simulink model "sistema_fisico_completo"  (R2023b)
settings: Solver=VariableStepAuto  StartTime=0.0  StopTime=10.0  RelTol=1e-3
undefined symbols (not defined in the file): b_cx, b_cy, b_hb, b_hEb, b_hwu, b_t, b_tb, b_tw, bh_eq, bt_eq, CI, g, H_c, i_h, i_t, Jh_eq, Jt_eq, K_cy, K_hwu, K_tw, L_h0, M_s, m_t, r_hd, r_td, T_hb_max, T_hEb_max, T_tb_max, Y_t0
settings Model: Creator=Ferran  LastModifiedBy=Ferran

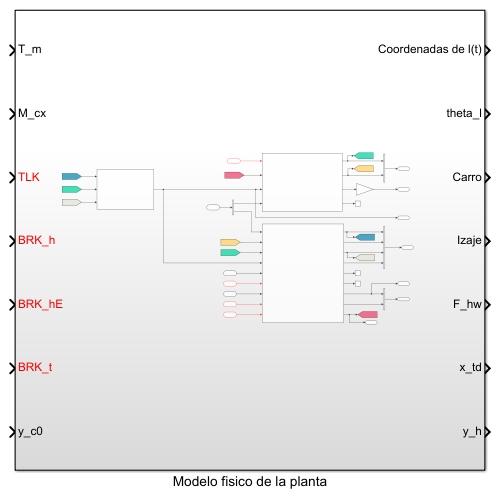
[thumbnail: Simulink's stored preview of the top-level diagram]
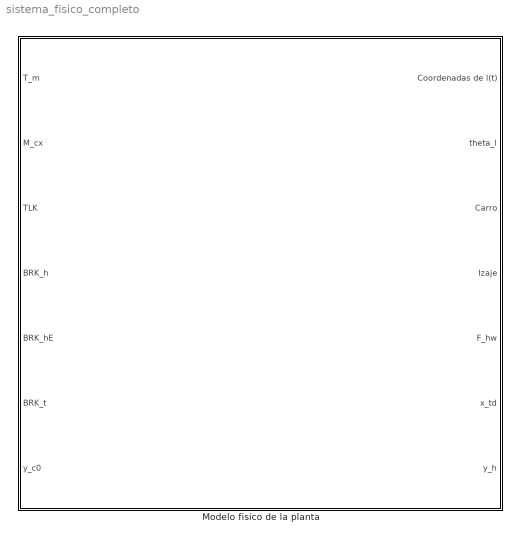
== system sistema_fisico_completo ==
  Modelo fisico de la planta : Subsystem

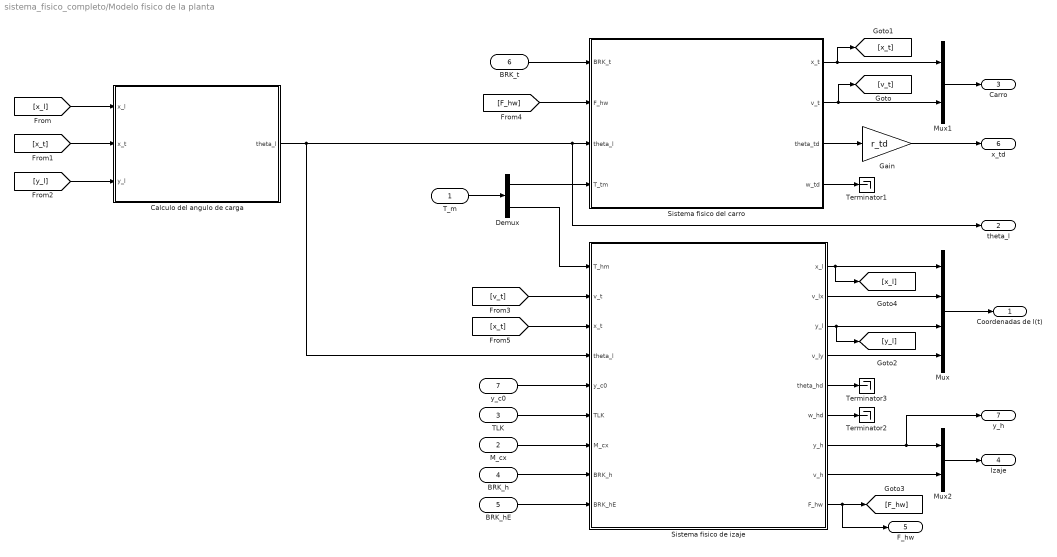
== system sistema_fisico_completo/Modelo fisico de la planta ==
  T_m : Inport
  M_cx : Inport  Port=2
  TLK : Inport  Port=3
  BRK_h : Inport  Port=4
  BRK_hE : Inport  Port=5
  BRK_t : Inport  Port=6
  y_c0 : Inport  Port=7
  Calculo del angulo de carga : Subsystem
  Demux : Demux  Outputs=2
  Gain : Gain  Gain=r_td
  Mux : Mux
  Mux1 : Mux  Inputs=2
  Mux2 : Mux  Inputs=2
  Sistema fisico de izaje : Subsystem
  Sistema fisico del carro : Subsystem
  Terminator1 : Terminator
  Terminator2 : Terminator
  Terminator3 : Terminator
  Coordenadas de l(t) : Outport
  theta_l : Outport  Port=2
  Carro : Outport  Port=3
  Izaje : Outport  Port=4
  F_hw : Outport  Port=5
  x_td : Outport  Port=6
  y_h : Outport  Port=7
  wires:
  [x_l] -> Calculo del angulo de carga/1(x_l)
  Sistema fisico del carro/3(theta_td) -> Gain/1
  Calculo del angulo de carga/1(theta_l) -> Sistema fisico del carro/3(theta_l), theta_l/1, Sistema fisico de izaje/4(theta_l)
  Sistema fisico de izaje/2(v_lx) -> Mux/2
  [x_t] -> Calculo del angulo de carga/2(x_t)
  y_c0/1 -> Sistema fisico de izaje/5(y_c0)
  Sistema fisico del carro/1(x_t) -> Mux1/1, [x_t]
  Sistema fisico de izaje/1(x_l) -> Mux/1, [x_l]
  Sistema fisico del carro/4(w_td) -> Terminator1/1
  [y_l] -> Calculo del angulo de carga/3(y_l)
  Sistema fisico de izaje/3(y_l) -> Mux/3, [y_l]
  [v_t] -> Sistema fisico de izaje/2(v_t)
  [x_t] -> Sistema fisico de izaje/3(x_t)
  Sistema fisico del carro/2(v_t) -> Mux1/2, [v_t]
  BRK_hE/1 -> Sistema fisico de izaje/9(BRK_hE)
  M_cx/1 -> Sistema fisico de izaje/7(M_cx)
  BRK_h/1 -> Sistema fisico de izaje/8(BRK_h)
  TLK/1 -> Sistema fisico de izaje/6(TLK)
  Demux/2 -> Sistema fisico de izaje/1(T_hm)
  [F_hw] -> Sistema fisico del carro/2(F_hw)
  Sistema fisico de izaje/9(F_hw) -> F_hw/1, [F_hw]
  Sistema fisico de izaje/4(v_ly) -> Mux/4
  Mux/1 -> Coordenadas de l(t)/1
  Mux1/1 -> Carro/1
  Sistema fisico de izaje/8(v_h) -> Mux2/2
  Mux2/1 -> Izaje/1
  Sistema fisico de izaje/5(theta_hd) -> Terminator3/1
  Sistema fisico de izaje/6(w_hd) -> Terminator2/1
  BRK_t/1 -> Sistema fisico del carro/1(BRK_t)
  Demux/1 -> Sistema fisico del carro/4(T_tm)
  T_m/1 -> Demux/1
  Sistema fisico de izaje/7(y_h) -> y_h/1, Mux2/1
  Gain/1 -> x_td/1

== system sistema_fisico_completo/Modelo fisico de la planta/Calculo del angulo de carga ==
  x_l : Inport
  x_t : Inport  Port=2
  y_l : Inport  Port=3
  Atan2 : Trigonometry  Operator=atan2
  Constant : Constant  Value=Y_t0
  Sum : Sum  Inputs=+-
  Sum1 : Sum  Inputs=+-
  theta_l : Outport
  wires:
  x_t/1 -> Sum/2
  Sum1/1 -> Atan2/2
  x_l/1 -> Sum/1
  Sum/1 -> Atan2/1
  Atan2/1 -> theta_l/1
  y_l/1 -> Sum1/2
  Constant/1 -> Sum1/1

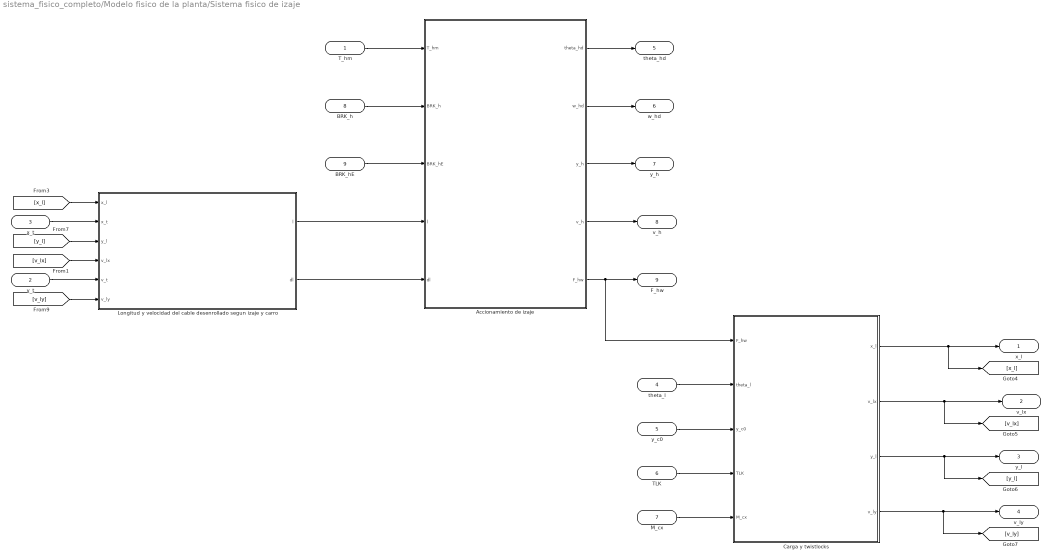
== system sistema_fisico_completo/Modelo fisico de la planta/Sistema fisico de izaje ==
  T_hm : Inport
  v_t : Inport  Port=2
  x_t : Inport  Port=3
  theta_l : Inport  Port=4
  y_c0 : Inport  Port=5
  TLK : Inport  Port=6
  M_cx : Inport  Port=7
  BRK_h : Inport  Port=8
  BRK_hE : Inport  Port=9
  Accionamiento de izaje : Subsystem
  Carga y twistlocks : Subsystem
  Longitud y velocidad del cable desenrollado segun izaje y carro : Subsystem
  x_l : Outport
  v_lx : Outport  Port=2
  y_l : Outport  Port=3
  v_ly : Outport  Port=4
  theta_hd : Outport  Port=5
  w_hd : Outport  Port=6
  y_h : Outport  Port=7
  v_h : Outport  Port=8
  F_hw : Outport  Port=9
  wires:
  [y_l] -> Longitud y velocidad del cable desenrollado segun izaje y carro/3(y_l)
  Accionamiento de izaje/5(F_hw) -> F_hw/1, Carga y twistlocks/1(F_hw)
  BRK_hE/1 -> Accionamiento de izaje/3(BRK_hE)
  Carga y twistlocks/1(x_l) -> x_l/1, [x_l]
  Carga y twistlocks/4(v_ly) -> v_ly/1, [v_ly]
  Accionamiento de izaje/3(y_h) -> y_h/1
  Carga y twistlocks/2(v_lx) -> v_lx/1, [v_lx]
  Longitud y velocidad del cable desenrollado segun izaje y carro/1(l) -> Accionamiento de izaje/4(l)
  Carga y twistlocks/3(y_l) -> y_l/1, [y_l]
  [v_lx] -> Longitud y velocidad del cable desenrollado segun izaje y carro/4(v_lx)
  [v_ly] -> Longitud y velocidad del cable desenrollado segun izaje y carro/6(v_ly)
  TLK/1 -> Carga y twistlocks/4(TLK)
  [x_l] -> Longitud y velocidad del cable desenrollado segun izaje y carro/1(x_l)
  T_hm/1 -> Accionamiento de izaje/1(T_hm)
  Accionamiento de izaje/1(theta_hd) -> theta_hd/1
  y_c0/1 -> Carga y twistlocks/3(y_c0)
  BRK_h/1 -> Accionamiento de izaje/2(BRK_h)
  Longitud y velocidad del cable desenrollado segun izaje y carro/2(dl) -> Accionamiento de izaje/5(dl)
  v_t/1 -> Longitud y velocidad del cable desenrollado segun izaje y carro/5(v_t)
  Accionamiento de izaje/4(v_h) -> v_h/1
  theta_l/1 -> Carga y twistlocks/2(theta_l)
  Accionamiento de izaje/2(w_hd) -> w_hd/1
  M_cx/1 -> Carga y twistlocks/5(M_cx)
  x_t/1 -> Longitud y velocidad del cable desenrollado segun izaje y carro/2(x_t)

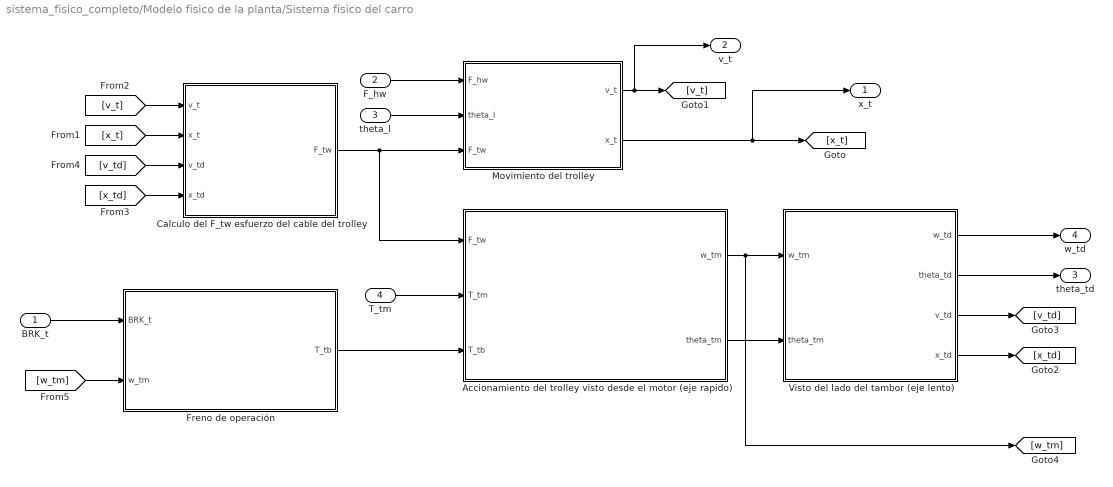
== system sistema_fisico_completo/Modelo fisico de la planta/Sistema fisico del carro ==
  BRK_t : Inport
  F_hw : Inport  Port=2
  theta_l : Inport  Port=3
  T_tm : Inport  Port=4
  Accionamiento del trolley visto desde el motor (eje rapido) : Subsystem
  Calculo del F_tw esfuerzo del cable del trolley : Subsystem
  Freno de operación : Subsystem
  Movimiento del trolley : Subsystem
  Visto del lado del tambor (eje lento) : Subsystem
  x_t : Outport
  v_t : Outport  Port=2
  theta_td : Outport  Port=3
  w_td : Outport  Port=4
  wires:
  [v_t] -> Calculo del F_tw esfuerzo del cable del trolley/1(v_t)
  Visto del lado del tambor (eje lento)/3(v_td) -> [v_td]
  Freno de operación/1(T_tb) -> Accionamiento del trolley visto desde el motor (eje rapido)/3(T_tb)
  Movimiento del trolley/1(v_t) -> v_t/1, [v_t]
  Movimiento del trolley/2(x_t) -> x_t/1, [x_t]
  Visto del lado del tambor (eje lento)/2(theta_td) -> theta_td/1
  BRK_t/1 -> Freno de operación/1(BRK_t)
  [w_tm] -> Freno de operación/2(w_tm)
  Accionamiento del trolley visto desde el motor (eje rapido)/1(w_tm) -> [w_tm], Visto del lado del tambor (eje lento)/1(w_tm)
  [x_td] -> Calculo del F_tw esfuerzo del cable del trolley/4(x_td)
  Accionamiento del trolley visto desde el motor (eje rapido)/2(theta_tm) -> Visto del lado del tambor (eje lento)/2(theta_tm)
  [x_t] -> Calculo del F_tw esfuerzo del cable del trolley/2(x_t)
  [v_td] -> Calculo del F_tw esfuerzo del cable del trolley/3(v_td)
  theta_l/1 -> Movimiento del trolley/2(theta_l)
  Visto del lado del tambor (eje lento)/4(x_td) -> [x_td]
  T_tm/1 -> Accionamiento del trolley visto desde el motor (eje rapido)/2(T_tm)
  Calculo del F_tw esfuerzo del cable del trolley/1(F_tw) -> Accionamiento del trolley visto desde el motor (eje rapido)/1(F_tw), Movimiento del trolley/3(F_tw)
  F_hw/1 -> Movimiento del trolley/1(F_hw)
  Visto del lado del tambor (eje lento)/1(w_td) -> w_td/1

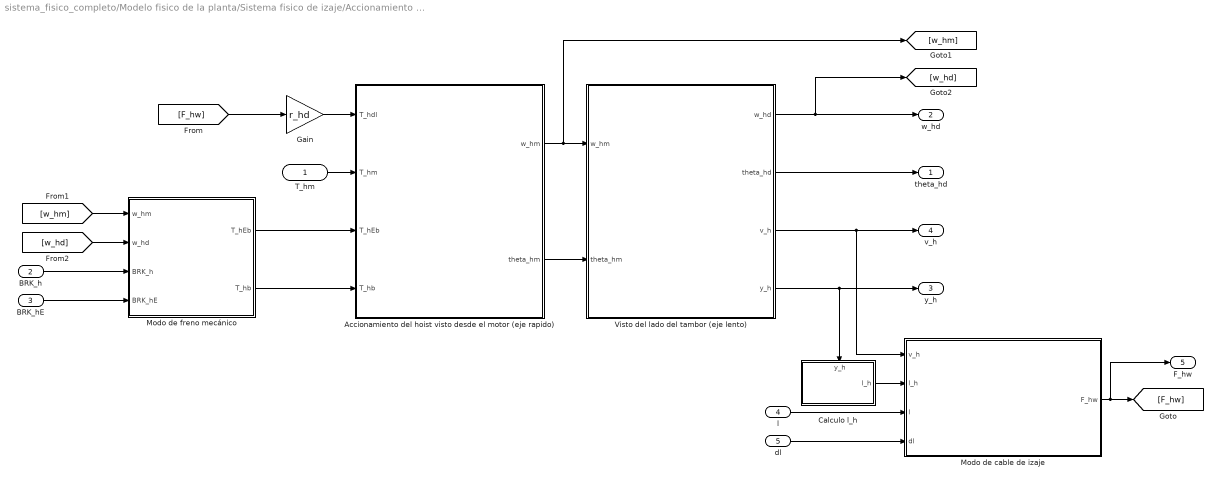
== system sistema_fisico_completo/Modelo fisico de la planta/Sistema fisico de izaje/Accionamiento de izaje ==
  T_hm : Inport
  BRK_h : Inport  Port=2
  BRK_hE : Inport  Port=3
  l : Inport  Port=4
  dl : Inport  Port=5
  Accionamiento del hoist visto desde el motor (eje rapido) : Subsystem
  Calculo l_h : Subsystem
      settings: PortSchema="{\"entries\":[{\"content\":{\"sides\":[{\"content\":{\"connectorIds\":[\"Out1\"]},\"type\":\"ConnectorPlacement.EquallySpacedRectSide\",\"uuid\":\"07ea2d8b-a4bd-4a00-9f3e-d3723522cead\"},{\"content\":{\"side\":\"RIGHT\"},\"type\":\"ConnectorPlacement.EquallySpacedRectSide\",\"uuid\":\"e7371649-c13b-4c3e-a52c-6db8f2f471a9\"},{\"content\":{\"side\":\"TOP\"},\"type\":\"ConnectorPlacement.EquallySpacedRectSide\",\"uuid\":\"bf44ddc9-8ab8-43a2-b974-62ce3b2d20dc\"},{\"content\":{\"connectorIds\":[\"In1\"],\"side\":\"BOTTOM\"},\"type\":\"ConnectorPlacement.EquallySpacedRectSide\",\"uuid\":\"68df679a-1ec0-4ce0-a9ee-39677e661654\"}]},\"type\":\"ConnectorPlacement.EquallySpacedConnector\",\"uuid\":\"345e5710-5df9-4bf4-96c9-62f27951d1e0\"}],\"packageUris\":[\"http://schema.mathworks.com/mf0/Connector/R2020b\"],\"version\":\"1.0\"}"
  Gain : Gain  Gain=r_hd
  Modo de cable de izaje : Subsystem
  Modo de freno mecánico : Subsystem
  Visto del lado del tambor (eje lento) : Subsystem
  theta_hd : Outport
  w_hd : Outport  Port=2
  y_h : Outport  Port=3
  v_h : Outport  Port=4
  F_hw : Outport  Port=5
  wires:
  Gain/1 -> Accionamiento del hoist visto desde el motor (eje rapido)/1(T_hdl)
  Accionamiento del hoist visto desde el motor (eje rapido)/1(w_hm) -> Visto del lado del tambor (eje lento)/1(w_hm), [w_hm]
  Visto del lado del tambor (eje lento)/1(w_hd) -> w_hd/1, [w_hd]
  Accionamiento del hoist visto desde el motor (eje rapido)/2(theta_hm) -> Visto del lado del tambor (eje lento)/2(theta_hm)
  dl/1 -> Modo de cable de izaje/4(dl)
  l/1 -> Modo de cable de izaje/3(l)
  [F_hw] -> Gain/1
  BRK_hE/1 -> Modo de freno mecánico/4(BRK_hE)
  Visto del lado del tambor (eje lento)/4(y_h) -> y_h/1, Calculo l_h/1(y_h)
  BRK_h/1 -> Modo de freno mecánico/3(BRK_h)
  Visto del lado del tambor (eje lento)/3(v_h) -> v_h/1, Modo de cable de izaje/1(v_h)
  Visto del lado del tambor (eje lento)/2(theta_hd) -> theta_hd/1
  T_hm/1 -> Accionamiento del hoist visto desde el motor (eje rapido)/2(T_hm)
  [w_hd] -> Modo de freno mecánico/2(w_hd)
  [w_hm] -> Modo de freno mecánico/1(w_hm)
  Calculo l_h/1(l_h) -> Modo de cable de izaje/2(l_h)
  Modo de freno mecánico/2(T_hb) -> Accionamiento del hoist visto desde el motor (eje rapido)/4(T_hb)
  Modo de cable de izaje/1(F_hw) -> F_hw/1, [F_hw]
  Modo de freno mecánico/1(T_hEb) -> Accionamiento del hoist visto desde el motor (eje rapido)/3(T_hEb)

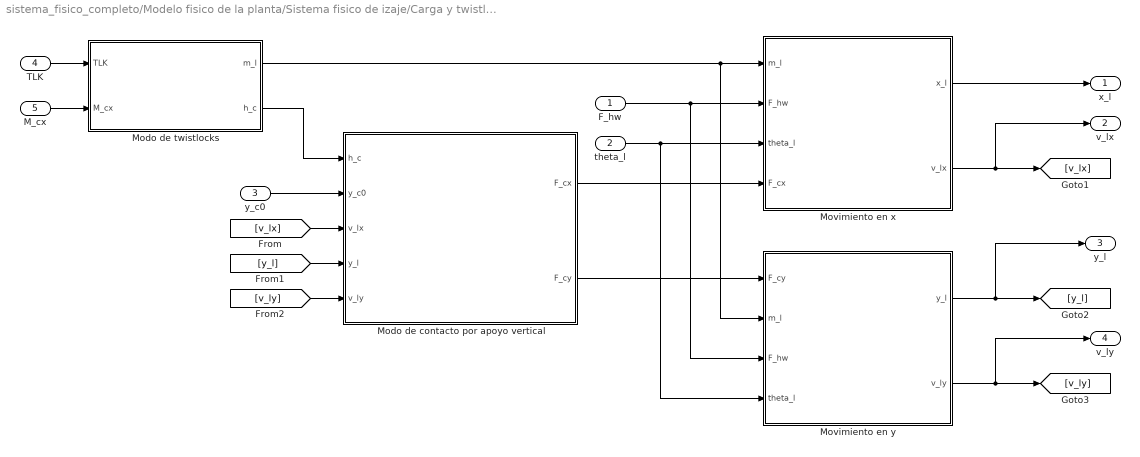
== system sistema_fisico_completo/Modelo fisico de la planta/Sistema fisico de izaje/Carga y twistlocks ==
  F_hw : Inport
  theta_l : Inport  Port=2
  y_c0 : Inport  Port=3
  TLK : Inport  Port=4
  M_cx : Inport  Port=5
  Modo de contacto por apoyo vertical : Subsystem
  Modo de twistlocks : Subsystem
  Movimiento en x : Subsystem
  Movimiento en y : Subsystem
  x_l : Outport
  v_lx : Outport  Port=2
  y_l : Outport  Port=3
  v_ly : Outport  Port=4
  wires:
  theta_l/1 -> Movimiento en y/4(theta_l), Movimiento en x/3(theta_l)
  Movimiento en y/2(v_ly) -> v_ly/1, [v_ly]
  y_c0/1 -> Modo de contacto por apoyo vertical/2(y_c0)
  Modo de contacto por apoyo vertical/2(F_cy) -> Movimiento en y/1(F_cy)
  [y_l] -> Modo de contacto por apoyo vertical/4(y_l)
  [v_lx] -> Modo de contacto por apoyo vertical/3(v_lx)
  Movimiento en x/2(v_lx) -> v_lx/1, [v_lx]
  TLK/1 -> Modo de twistlocks/1(TLK)
  Movimiento en x/1(x_l) -> x_l/1
  Modo de twistlocks/1(m_l) -> Movimiento en x/1(m_l), Movimiento en y/2(m_l)
  [v_ly] -> Modo de contacto por apoyo vertical/5(v_ly)
  Movimiento en y/1(y_l) -> y_l/1, [y_l]
  Modo de contacto por apoyo vertical/1(F_cx) -> Movimiento en x/4(F_cx)
  F_hw/1 -> Movimiento en y/3(F_hw), Movimiento en x/2(F_hw)
  M_cx/1 -> Modo de twistlocks/2(M_cx)
  Modo de twistlocks/2(h_c) -> Modo de contacto por apoyo vertical/1(h_c)

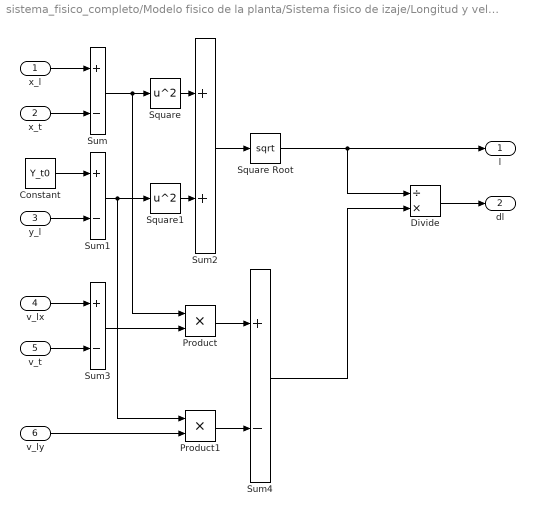
== system sistema_fisico_completo/Modelo fisico de la planta/Sistema fisico de izaje/Longitud y velocidad del cable desenrollado segun izaje y carro ==
  x_l : Inport
  x_t : Inport  Port=2
  y_l : Inport  Port=3
  v_lx : Inport  Port=4
  v_t : Inport  Port=5
  v_ly : Inport  Port=6
  Constant : Constant  Value=Y_t0
  Divide : Product  Inputs=/*
  Product : Product
  Product1 : Product
  Square : Math  Operator=square
  Square Root : Sqrt
  Square1 : Math  Operator=square
  Sum{,1,3..4} (4 alike) : Sum  Inputs=+-
  Sum2 : Sum
  l : Outport
  dl : Outport  Port=2
  wires:
  Sum/1 -> Product/1, Square/1
  Divide/1 -> dl/1
  Product1/1 -> Sum4/2
  Sum3/1 -> Product/2
  Product/1 -> Sum4/1
  Square Root/1 -> l/1, Divide/1
  Constant/1 -> Sum1/1
  Sum4/1 -> Divide/2
  y_l/1 -> Sum1/2
  x_l/1 -> Sum/1
  Square1/1 -> Sum2/2
  v_t/1 -> Sum3/2
  Sum1/1 -> Square1/1, Product1/1
  v_ly/1 -> Product1/2
  Square/1 -> Sum2/1
  v_lx/1 -> Sum3/1
  x_t/1 -> Sum/2
  Sum2/1 -> Square Root/1

== system sistema_fisico_completo/Modelo fisico de la planta/Sistema fisico del carro/Accionamiento del trolley visto desde el motor (eje rapido) ==
  F_tw : Inport
  T_tm : Inport  Port=2
  T_tb : Inport  Port=3
  Gain : Gain  Gain=r_td / i_t
  Integrator : Integrator  InitialCondition=CI(1) * (i_t / r_td)
  Integrator1 : Integrator
  Momento de inercia del trolley equivalente : Gain  Gain=1 / Jt_eq
  Sum : Sum  Inputs=--++
  Viscosidad del trolley equivalente : Gain  Gain=bt_eq
  w_tm : Outport
  theta_tm : Outport  Port=2
  wires:
  Gain/1 -> Sum/2
  Integrator/1 -> theta_tm/1
  Sum/1 -> Momento de inercia del trolley equivalente/1
  Integrator1/1 -> Viscosidad del trolley equivalente/1, w_tm/1, Integrator/1  "w_tm"
  Viscosidad del trolley equivalente/1 -> Sum/1
  Momento de inercia del trolley equivalente/1 -> Integrator1/1  "dw_tm"
  F_tw/1 -> Gain/1
  T_tb/1 -> Sum/4
  T_tm/1 -> Sum/3

== system sistema_fisico_completo/Modelo fisico de la planta/Sistema fisico del carro/Calculo del F_tw esfuerzo del cable del trolley ==
  v_t : Inport
  x_t : Inport  Port=2
  v_td : Inport  Port=3
  x_td : Inport  Port=4
  Gain : Gain  Gain=K_tw
  Gain1 : Gain  Gain=b_tw
  Sum : Sum  Inputs=+-
  Sum2 : Sum  Inputs=+-
  Sum3 : Sum
  F_tw : Outport
  wires:
  x_td/1 -> Sum/1
  Sum/1 -> Gain/1
  v_td/1 -> Sum2/1
  Sum2/1 -> Gain1/1
  v_t/1 -> Sum2/2
  x_t/1 -> Sum/2
  Sum3/1 -> F_tw/1
  Gain/1 -> Sum3/1
  Gain1/1 -> Sum3/2

== system sistema_fisico_completo/Modelo fisico de la planta/Sistema fisico del carro/Freno de operación ==
  note: Si BRK_t = 0 (Off - desenergizado) ... entonces ... T_tb != 0
      | Si BRK_t = 1 (On - energizado) ... entonces ... T_tb == 0
  BRK_t : Inport
  w_tm : Inport  Port=2
  Constant1 : Constant  Value=-T_tb_max
  Constant2 : Constant  Value=T_tb_max
  Flip : Subsystem
  Gain : Gain  Gain=- b_tb
  Max : MinMax  Function=max  Inputs=2
  Min : MinMax  Inputs=2
  Product : Product
  T_tb : Outport
  wires:
  Constant1/1 -> Max/1
  w_tm/1 -> Gain/1
  Max/1 -> Min/2
  BRK_t/1 -> Flip/1(BRK_t)
  Min/1 -> Product/2
  Product/1 -> T_tb/1
  Constant2/1 -> Min/1
  Gain/1 -> Max/2
  Flip/1(Out1) -> Product/1

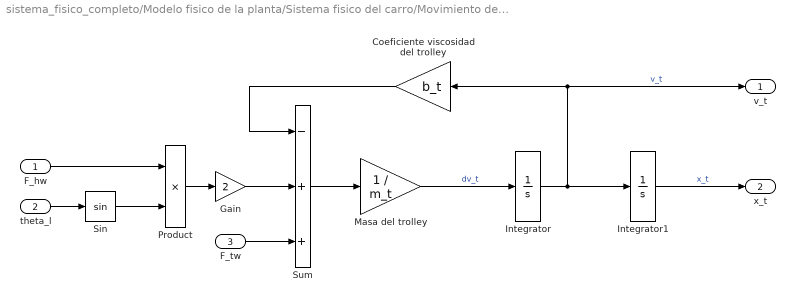
== system sistema_fisico_completo/Modelo fisico de la planta/Sistema fisico del carro/Movimiento del trolley ==
  F_hw : Inport
  theta_l : Inport  Port=2
  F_tw : Inport  Port=3
  Coeficiente viscosidad del trolley : Gain  Gain=b_t
  Gain : Gain  Gain=2
  Integrator : Integrator
  Integrator1 : Integrator  InitialCondition=CI(1)
  Masa del trolley : Gain  Gain=1 / m_t
  Product : Product
  Sin : Trigonometry
  Sum : Sum  Inputs=-++
  v_t : Outport
  x_t : Outport  Port=2
  wires:
  Sin/1 -> Product/2
  F_tw/1 -> Sum/3
  Integrator/1 -> v_t/1, Coeficiente viscosidad del trolley/1, Integrator1/1  "v_t"
  F_hw/1 -> Product/1
  Integrator1/1 -> x_t/1  "x_t"
  Product/1 -> Gain/1
  Sum/1 -> Masa del trolley/1
  theta_l/1 -> Sin/1
  Masa del trolley/1 -> Integrator/1  "dv_t"
  Gain/1 -> Sum/2
  Coeficiente viscosidad del trolley/1 -> Sum/1

== system sistema_fisico_completo/Modelo fisico de la planta/Sistema fisico del carro/Visto del lado del tambor (eje lento) ==
  w_tm : Inport
  theta_tm : Inport  Port=2
  Gain : Gain  Gain=1 / i_t
  Gain1 : Gain  Gain=1 / i_t
  r_td : Gain  Gain=r_td
  r_td1 : Gain  Gain=r_td
  w_td : Outport
  theta_td : Outport  Port=2
  v_td : Outport  Port=3
  x_td : Outport  Port=4
  wires:
  Gain1/1 -> r_td1/1, theta_td/1
  Gain/1 -> w_td/1, r_td/1
  w_tm/1 -> Gain/1
  theta_tm/1 -> Gain1/1
  r_td/1 -> v_td/1
  r_td1/1 -> x_td/1

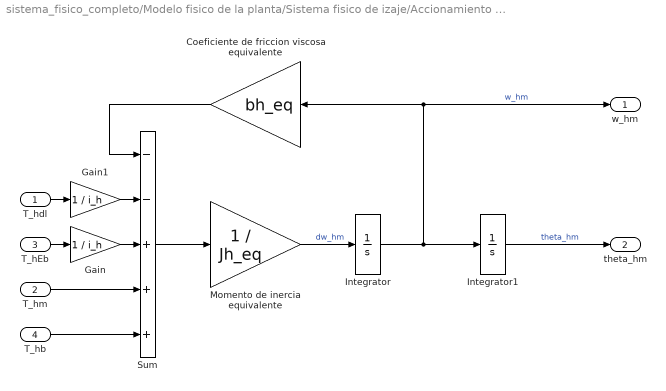
== system sistema_fisico_completo/Modelo fisico de la planta/Sistema fisico de izaje/Accionamiento de izaje/Accionamiento del hoist visto desde el motor (eje rapido) ==
  T_hdl : Inport
  T_hm : Inport  Port=2
  T_hEb : Inport  Port=3
  T_hb : Inport  Port=4
  Coeficiente de friccion viscosa equivalente : Gain  Gain=bh_eq
  Gain : Gain  Gain=1 / i_h
  Gain1 : Gain  Gain=1 / i_h
  Integrator : Integrator
  Integrator1 : Integrator  InitialCondition=CI(3) * ((2 * i_h)/ r_hd)
  Momento de inercia equivalente : Gain  Gain=1 / Jh_eq
  Sum : Sum  Inputs=--+++
  w_hm : Outport
  theta_hm : Outport  Port=2
  wires:
  Integrator1/1 -> theta_hm/1  "theta_hm"
  Coeficiente de friccion viscosa equivalente/1 -> Sum/1
  T_hm/1 -> Sum/4
  Momento de inercia equivalente/1 -> Integrator/1  "dw_hm"
  T_hEb/1 -> Gain/1
  Integrator/1 -> Coeficiente de friccion viscosa equivalente/1, w_hm/1, Integrator1/1  "w_hm"
  T_hb/1 -> Sum/5
  Sum/1 -> Momento de inercia equivalente/1
  T_hdl/1 -> Gain1/1
  Gain/1 -> Sum/3
  Gain1/1 -> Sum/2

== system sistema_fisico_completo/Modelo fisico de la planta/Sistema fisico de izaje/Accionamiento de izaje/Calculo l_h ==
  y_h : Inport
  Constant : Constant  Value=Y_t0
  Sum : Sum  Inputs=+-
  l_h : Outport
  wires:
  Constant/1 -> Sum/1
  Sum/1 -> l_h/1
  y_h/1 -> Sum/2

== system sistema_fisico_completo/Modelo fisico de la planta/Sistema fisico de izaje/Accionamiento de izaje/Modo de cable de izaje ==
  note: El bloque if analiza cual bloque de accion se habilita (action subsystem), luego se usa el bloque merge para unir las salidas y determinar la salida final segun se haya decidido desde el bloque if
      |
      | En este caso el modo de cable:
      | cuando l(t) >= l_h(t) entonces esta tensado
      | cuando l(t) < l_h(t) entonces esta flojo
  v_h : Inport
  l_h : Inport  Port=2
  l : Inport  Port=3
  dl : Inport  Port=4
  Cable flojo : Subsystem  TreatAsAtomicUnit=on
  Cable tensado : Subsystem  TreatAsAtomicUnit=on
  Decision del modo de cable de izaje : If  NumInputs=2  IfExpression=u2 >= u1
  Merge : Merge
  F_hw : Outport
  wires:
  Decision del modo de cable de izaje/1 -> Cable tensado/Action
  Decision del modo de cable de izaje/2 -> Cable flojo/Action
  l/1 -> Decision del modo de cable de izaje/2, Cable tensado/2(l)
  Cable flojo/1(Out1) -> Merge/2
  dl/1 -> Cable tensado/4(dl)
  l_h/1 -> Decision del modo de cable de izaje/1, Cable tensado/1(l_h)
  Cable tensado/1(F_hw) -> Merge/1
  v_h/1 -> Cable tensado/3(v_h)
  Merge/1 -> F_hw/1

== system sistema_fisico_completo/Modelo fisico de la planta/Sistema fisico de izaje/Accionamiento de izaje/Modo de freno mecánico ==
  w_hm : Inport
  w_hd : Inport  Port=2
  BRK_h : Inport  Port=3
  BRK_hE : Inport  Port=4
  Freno de emergencia : Subsystem
  Freno de operación : Subsystem
  T_hEb : Outport
  T_hb : Outport  Port=2
  wires:
  w_hm/1 -> Freno de operación/2(w_hm)
  BRK_hE/1 -> Freno de emergencia/1(BRK_hE)
  Freno de operación/1(T_hb) -> T_hb/1
  Freno de emergencia/1(T_hEb) -> T_hEb/1
  w_hd/1 -> Freno de emergencia/2(w_hd)
  BRK_h/1 -> Freno de operación/1(BRK_h)

== system sistema_fisico_completo/Modelo fisico de la planta/Sistema fisico de izaje/Accionamiento de izaje/Visto del lado del tambor (eje lento) ==
  w_hm : Inport
  theta_hm : Inport  Port=2
  Gain : Gain  Gain=1 / i_h
  Gain1 : Gain  Gain=1 / i_h
  r_td : Gain  Gain=r_hd / 2
  r_td1 : Gain  Gain=r_hd / 2
  w_hd : Outport
  theta_hd : Outport  Port=2
  v_h : Outport  Port=3
  y_h : Outport  Port=4
  wires:
  Gain1/1 -> r_td1/1, theta_hd/1
  Gain/1 -> w_hd/1, r_td/1
  w_hm/1 -> Gain/1
  theta_hm/1 -> Gain1/1
  r_td/1 -> v_h/1
  r_td1/1 -> y_h/1

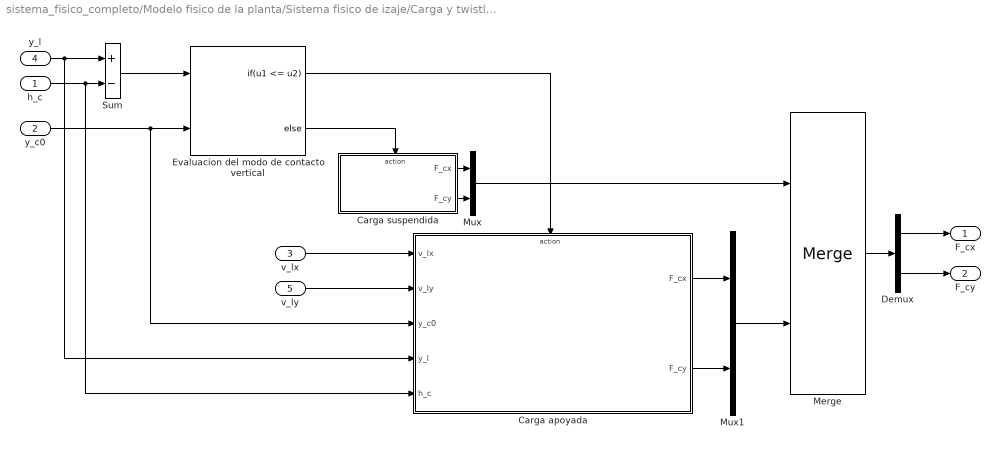
== system sistema_fisico_completo/Modelo fisico de la planta/Sistema fisico de izaje/Carga y twistlocks/Modo de contacto por apoyo vertical ==
  h_c : Inport
  y_c0 : Inport  Port=2
  v_lx : Inport  Port=3
  y_l : Inport  Port=4
  v_ly : Inport  Port=5
  Carga apoyada : Subsystem  TreatAsAtomicUnit=on
  Carga suspendida : Subsystem  TreatAsAtomicUnit=on
  Demux : Demux  Outputs=2
  Evaluacion del modo de contacto vertical : If  NumInputs=2  IfExpression=u1 <= u2
  Merge : Merge
  Mux : Mux  Inputs=2
  Mux1 : Mux  Inputs=2
  Sum : Sum  Inputs=+-
  F_cx : Outport
  F_cy : Outport  Port=2
  wires:
  Carga apoyada/2(F_cy) -> Mux1/2
  Evaluacion del modo de contacto vertical/1 -> Carga apoyada/Action
  Evaluacion del modo de contacto vertical/2 -> Carga suspendida/Action
  y_c0/1 -> Carga apoyada/3(y_c0), Evaluacion del modo de contacto vertical/2
  v_lx/1 -> Carga apoyada/1(v_lx)
  Sum/1 -> Evaluacion del modo de contacto vertical/1
  y_l/1 -> Carga apoyada/4(y_l), Sum/1
  h_c/1 -> Sum/2, Carga apoyada/5(h_c)
  Carga suspendida/1(F_cx) -> Mux/1
  Carga suspendida/2(F_cy) -> Mux/2
  Mux/1 -> Merge/1
  Carga apoyada/1(F_cx) -> Mux1/1
  Mux1/1 -> Merge/2
  Merge/1 -> Demux/1
  Demux/1 -> F_cx/1
  Demux/2 -> F_cy/1
  v_ly/1 -> Carga apoyada/2(v_ly)

== system sistema_fisico_completo/Modelo fisico de la planta/Sistema fisico de izaje/Carga y twistlocks/Modo de twistlocks ==
  note: Si TLK = 0 (Off) ... entonces ... h_c = 0
      | Si TLK = 1 (On) ... entonces ... h_c = H_c
  note: Si TLK = 0 (Off) ... entonces ... m_l = M_s
      | Si TLK = 1 (On) ... entonces ... m_l = M_s + M_cx
  TLK : Inport
  M_cx : Inport  Port=2
  Altura del container : Constant  Value=H_c
  Masa del spreader : Constant  Value=M_s
  Product : Product
  Product1 : Product
  Sum : Sum
  m_l : Outport
  h_c : Outport  Port=2
  wires:
  M_cx/1 -> Product/2
  Sum/1 -> m_l/1
  TLK/1 -> Product/1, Product1/1
  Masa del spreader/1 -> Sum/1
  Product/1 -> Sum/2
  Altura del container/1 -> Product1/2
  Product1/1 -> h_c/1

== system sistema_fisico_completo/Modelo fisico de la planta/Sistema fisico de izaje/Carga y twistlocks/Movimiento en x ==
  m_l : Inport
  F_hw : Inport  Port=2
  theta_l : Inport  Port=3
  F_cx : Inport  Port=4
  Divide : Product  Inputs=*/
  Gain : Gain  Gain=2
  Integrator : Integrator
  Integrator1 : Integrator
  Product : Product
  Sin : Trigonometry
  Sum : Sum  Inputs=-+
  x_l : Outport
  v_lx : Outport  Port=2
  wires:
  Integrator1/1 -> x_l/1
  Product/1 -> Sum/1
  Sum/1 -> Divide/1
  m_l/1 -> Divide/2
  Integrator/1 -> v_lx/1, Integrator1/1  "dx_l"
  Sin/1 -> Product/1
  theta_l/1 -> Sin/1
  F_cx/1 -> Sum/2
  Divide/1 -> Integrator/1  "ddx_l"
  F_hw/1 -> Gain/1
  Gain/1 -> Product/2

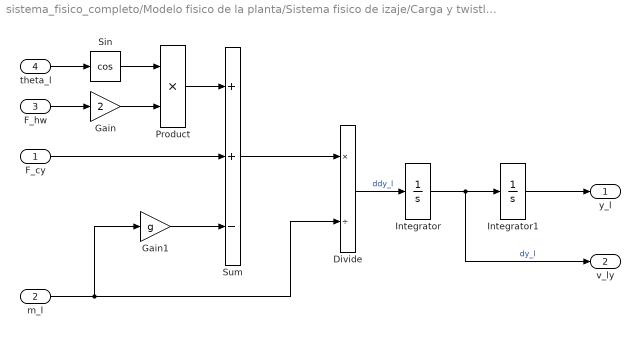
== system sistema_fisico_completo/Modelo fisico de la planta/Sistema fisico de izaje/Carga y twistlocks/Movimiento en y ==
  F_cy : Inport
  m_l : Inport  Port=2
  F_hw : Inport  Port=3
  theta_l : Inport  Port=4
  Divide : Product  Inputs=*/
  Gain : Gain  Gain=2
  Gain1 : Gain  Gain=g
  Integrator : Integrator
  Integrator1 : Integrator  InitialCondition=CI(3)
  Product : Product
  Sin : Trigonometry  Operator=cos
  Sum : Sum  Inputs=++-
  y_l : Outport
  v_ly : Outport  Port=2
  wires:
  Integrator1/1 -> y_l/1
  Product/1 -> Sum/1
  Sum/1 -> Divide/1
  m_l/1 -> Divide/2, Gain1/1
  Integrator/1 -> v_ly/1, Integrator1/1  "dy_l"
  Sin/1 -> Product/1
  theta_l/1 -> Sin/1
  F_cy/1 -> Sum/2
  Divide/1 -> Integrator/1  "ddy_l"
  F_hw/1 -> Gain/1
  Gain/1 -> Product/2
  Gain1/1 -> Sum/3

== system sistema_fisico_completo/Modelo fisico de la planta/Sistema fisico del carro/Freno de operación/Flip ==
  note: Como la decision de desenergizar (Off) representa un 0 pero a la salida existe un valor diferente de cero, se utiliza este sistema para cambiar el cero (0) por un uno (1).
      |
      | Esto es debido a que se usa el bloque de producto que multiplica la señal de BRK_t por el calculo pertinente a T_tb.
  BRK_t : Inport
  Constant : Constant  Value=[1 0]
  Selector : Selector  IndexMode=Zero-based  InputPortWidth=2  IndexOptions=Starting index (port)  Indices=[1 3]  OutputSizes=1
  Out1 : Outport
  wires:
  BRK_t/1 -> Selector/2
  Constant/1 -> Selector/1
  Selector/1 -> Out1/1

== system sistema_fisico_completo/Modelo fisico de la planta/Sistema fisico de izaje/Accionamiento de izaje/Modo de cable de izaje/Cable flojo ==
  Action Port : ActionPort
  Zero : Constant  Value=0  OutDataTypeStr=Inherit: Inherit via back propagation
  Out1 : Outport
  wires:
  Zero/1 -> Out1/1

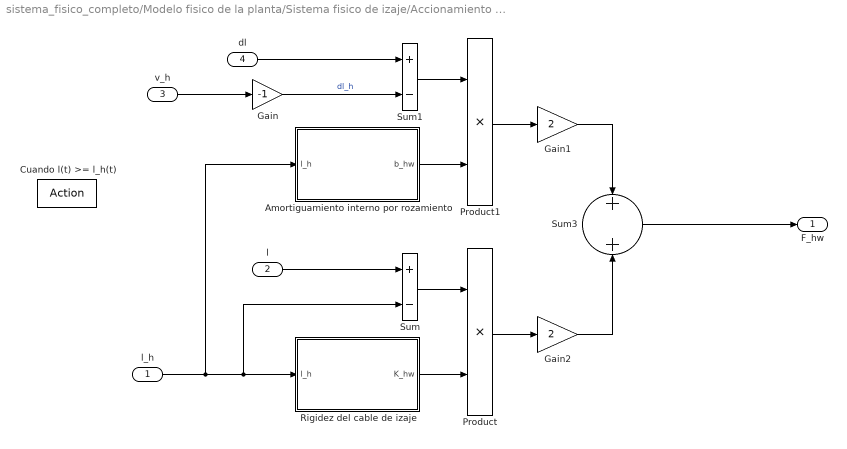
== system sistema_fisico_completo/Modelo fisico de la planta/Sistema fisico de izaje/Accionamiento de izaje/Modo de cable de izaje/Cable tensado ==
  l_h : Inport
  l : Inport  Port=2
  v_h : Inport  Port=3
  dl : Inport  Port=4
  Cuando l(t) >= l_h(t) : ActionPort
  Amortiguamiento interno por rozamiento : Subsystem
  Gain : Gain  Gain=-1
  Gain1 : Gain  Gain=2
  Gain2 : Gain  Gain=2
  Product : Product
  Product1 : Product
  Rigidez del cable de izaje : Subsystem
  Sum : Sum  Inputs=+-
  Sum1 : Sum  Inputs=+-
  Sum3 : Sum
  F_hw : Outport
  wires:
  l/1 -> Sum/1
  l_h/1 -> Amortiguamiento interno por rozamiento/1(l_h), Rigidez del cable de izaje/1(l_h), Sum/2
  Sum3/1 -> F_hw/1
  Gain1/1 -> Sum3/1
  Gain2/1 -> Sum3/2
  Rigidez del cable de izaje/1(K_hw) -> Product/2
  Amortiguamiento interno por rozamiento/1(b_hw) -> Product1/2
  Sum1/1 -> Product1/1
  Sum/1 -> Product/1
  v_h/1 -> Gain/1
  Product1/1 -> Gain1/1
  Product/1 -> Gain2/1
  dl/1 -> Sum1/1
  Gain/1 -> Sum1/2  "dl_h"

== system sistema_fisico_completo/Modelo fisico de la planta/Sistema fisico de izaje/Accionamiento de izaje/Modo de freno mecánico/Freno de emergencia ==
  note: Si BRK_h = 0 (Off - desenergizado) ... entonces ... T_hb != 0
      | Si BRK_h = 1 (On - energizado) ... entonces ... T_hb == 0
  BRK_hE : Inport
  w_hd : Inport  Port=2
  Flip : Subsystem
  Gain : Gain  Gain=- b_hEb
  Product : Product
  Saturation : Saturate  UpperLimit=T_hEb_max  LowerLimit=-T_hEb_max
  T_hEb : Outport
  wires:
  w_hd/1 -> Gain/1
  BRK_hE/1 -> Flip/1(BRK_hE)
  Product/1 -> T_hEb/1
  Gain/1 -> Saturation/1
  Flip/1(Out1) -> Product/1
  Saturation/1 -> Product/2

== system sistema_fisico_completo/Modelo fisico de la planta/Sistema fisico de izaje/Accionamiento de izaje/Modo de freno mecánico/Freno de operación ==
  note: Si BRK_h = 0 (Off - desenergizado) ... entonces ... T_hb != 0
      | Si BRK_h = 1 (On - energizado) ... entonces ... T_hb == 0
  BRK_h : Inport
  w_hm : Inport  Port=2
  Flip : Subsystem
  Gain : Gain  Gain=- b_hb
  Product : Product
  Saturation : Saturate  UpperLimit=T_hb_max  LowerLimit=-T_hb_max
  T_hb : Outport
  wires:
  w_hm/1 -> Gain/1
  BRK_h/1 -> Flip/1(BRK_h)
  Product/1 -> T_hb/1
  Flip/1(Out1) -> Product/1
  Saturation/1 -> Product/2
  Gain/1 -> Saturation/1

== system sistema_fisico_completo/Modelo fisico de la planta/Sistema fisico de izaje/Carga y twistlocks/Modo de contacto por apoyo vertical/Carga apoyada ==
  v_lx : Inport
  v_ly : Inport  Port=2
  y_c0 : Inport  Port=3
  y_l : Inport  Port=4
  h_c : Inport  Port=5
  Action Port : ActionPort
  Gain : Gain  Gain=- b_cx
  Gain1 : Gain  Gain=K_cy
  Gain2 : Gain  Gain=b_cy
  Sum : Sum  Inputs=+-
  Sum1 : Sum  Inputs=-++
  F_cx : Outport
  F_cy : Outport  Port=2
  wires:
  v_lx/1 -> Gain/1
  Gain/1 -> F_cx/1
  Gain1/1 -> Sum/1
  Sum/1 -> F_cy/1
  Gain2/1 -> Sum/2
  v_ly/1 -> Gain2/1
  Sum1/1 -> Gain1/1
  y_l/1 -> Sum1/1
  h_c/1 -> Sum1/2
  y_c0/1 -> Sum1/3

== system sistema_fisico_completo/Modelo fisico de la planta/Sistema fisico de izaje/Carga y twistlocks/Modo de contacto por apoyo vertical/Carga suspendida ==
  Action Port : ActionPort
  Zero : Constant  Value=0  OutDataTypeStr=Inherit: Inherit via back propagation
  F_cx : Outport
  F_cy : Outport  Port=2
  wires:
  Zero/1 -> F_cx/1, F_cy/1

== system sistema_fisico_completo/Modelo fisico de la planta/Sistema fisico de izaje/Accionamiento de izaje/Modo de cable de izaje/Cable tensado/Amortiguamiento interno por rozamiento ==
  l_h : Inport
  Constant : Constant  Value=L_h0
  Gain : Gain  Gain=2
  Gain1 : Gain  Gain=b_hwu
  Sum : Sum
  b_hw : Outport
  wires:
  Sum/1 -> Gain1/1
  Gain/1 -> Sum/1
  Gain1/1 -> b_hw/1
  Constant/1 -> Sum/2
  l_h/1 -> Gain/1

== system sistema_fisico_completo/Modelo fisico de la planta/Sistema fisico de izaje/Accionamiento de izaje/Modo de cable de izaje/Cable tensado/Rigidez del cable de izaje ==
  l_h : Inport
  Constant : Constant  Value=K_hwu
  Constant1 : Constant  Value=L_h0
  Divide : Product  Inputs=*/
  Gain : Gain  Gain=2
  Sum : Sum
  K_hw : Outport
  wires:
  Constant1/1 -> Sum/2
  Sum/1 -> Divide/2
  Gain/1 -> Sum/1
  Constant/1 -> Divide/1
  Divide/1 -> K_hw/1
  l_h/1 -> Gain/1

== system sistema_fisico_completo/Modelo fisico de la planta/Sistema fisico de izaje/Accionamiento de izaje/Modo de freno mecánico/Freno de emergencia/Flip ==
  note: Como la decision de desenergizar (Off) representa un 0 pero a la salida existe un valor diferente de cero, se utiliza este sistema para cambiar el cero (0) por un uno (1).
      |
      | Esto es debido a que se usa el bloque de producto que multiplica la señal de BRK_hE por el calculo pertinente a T_hEb.
  BRK_hE : Inport
  Constant : Constant  Value=[1 0]
  Selector : Selector  IndexMode=Zero-based  InputPortWidth=2  IndexOptions=Starting index (port)  Indices=[1 3]  OutputSizes=1
  Out1 : Outport
  wires:
  BRK_hE/1 -> Selector/2
  Constant/1 -> Selector/1
  Selector/1 -> Out1/1

== system sistema_fisico_completo/Modelo fisico de la planta/Sistema fisico de izaje/Accionamiento de izaje/Modo de freno mecánico/Freno de operación/Flip ==
  note: Como la decision de desenergizar (Off) representa un 0 pero a la salida existe un valor diferente de cero, se utiliza este sistema para cambiar el cero (0) por un uno (1).
      |
      | Esto es debido a que se usa el bloque de producto que multiplica la señal de BRK_h por el calculo pertinente a T_hb.
  BRK_h : Inport
  Constant : Constant  Value=[1 0]
  Selector : Selector  IndexMode=Zero-based  InputPortWidth=2  IndexOptions=Starting index (port)  Indices=[1 3]  OutputSizes=1
  Out1 : Outport
  wires:
  BRK_h/1 -> Selector/2
  Constant/1 -> Selector/1
  Selector/1 -> Out1/1
